simulink model "RejectDoublePress_Adhoc_Harness"  (R2019a)
settings: Solver=FixedStepDiscrete  StartTime=0.0  StopTime=Inf  FixedStep=0.1  RelTol=1e-3  EnableMultiTasking=on
settings Model: EnablePacing=on  Creator=colosky  LastModifiedBy=colosky
settings DataIOCC: LimitDataPoints=on  SaveFormat=Array  SaveOutput=off  SignalLogging=off  DSMLogging=off  SaveTime=off  ReturnWorkspaceOutputs=off
settings OptimizationCC: DefaultParameterBehavior=Inlined  InlineInvariantSignals=on  ExpressionDepthLimit=2147483647  InitFltsAndDblsToZero=on  NoFixptDivByZeroProtection=on  LifeSpan=inf
settings DebuggingCC: SignalInfNanChecking=warning  SaveWithParameterizedLinksMsg=none  UnderspecifiedInitializationDetection=Classic  MergeDetectMultiDrivingBlocksExec=none  SolverPrmCheckMsg=warning  FcnCallInpInsideContextMsg=warning  UniqueDataStoreMsg=warning  AllowSymbolicDim=off  StateNameClashWarn=warning  StrictBusMsg=ErrorOnBusTreatedAsVector  SFUnexpectedBacktrackingDiag=warning  SFNoUnconditionalDefaultTransitionDiag=warning  SFExecutionAtInitializationDiag=none  ArithmeticOperatorsInVariantConditions=warning
settings HardwareCC: ProdBitPerPointer=32  ProdBitPerSizeT=32  ProdBitPerPtrDiffT=32  ProdLargestAtomicFloat=None  ProdIntDivRoundTo=Undefined  ProdEndianess=Unspecified  ProdWordSize=32  ProdHWDeviceType=32-bit Generic
settings ModelReferenceCC: ModelReferenceNumInstancesAllowed=Single  PropagateSignalLabelsOutOfModel=off
settings SFSimCC: SimUseLocalCustomCode=off  SimParseCustomCode=off  MATLABDynamicMemAlloc=off
settings RTWCC: SystemTargetFile=ert.tlc  TemplateMakefile=ert_default_tmf  GenerateReport=on  RTWUseLocalCustomCode=off  IncludeHyperlinkInReport=on  LaunchReport=on  PortableWordSizes=on  GenerateTraceInfo=on  GenerateTraceReport=on  GenerateTraceReportSl=on  GenerateTraceReportSf=on  GenerateTraceReportEml=on
settings CodeAppCC: IgnoreCustomStorageClasses=off  CustomSymbolStrGlobalVar=$N$M  StateflowObjectComments=on
settings ERTTargetCC: MultiwordLength=2048  GenerateSampleERTMain=on  InlinedParameterPlacement=NonHierarchical  ERTCustomFileTemplate=example_file_process.tlc  ConvertIfToSwitch=off  SuppressUnreachableDefaultCases=off
settings ConfigComp: CovScope=ReferencedModels  CovMetricSettings=dcme  CovExternalEMLEnable=off  CovSFcnEnable=off  DVMode=DesignErrorDetection  DVMaxProcessTime=3000  DVDisplayUnsatisfiableObjectives=on  DVAutomaticStubbing=off  DVMakeOutputFilesUnique=off  DVParameters=on  DVParametersUseConfig=on  DVModelCoverageObjectives=MCDC  DVMaxTestCaseSteps=500  DVTestSuiteOptimization=CombinedObjectives  DVAssertions=EnableAll  DVProofAssumptions=EnableAll  DVIgnoreCovSatisfied=on  DVCoverageDataFile=CruiseControlCovManual.cvt  DVDetectDeadLogic=on  DVDetectActiveLogic=on  DVDetectIntegerOverflow=off  DVMaxViolationSteps=50  DVSaveDataFile=off  DVSaveHarnessModel=on  DVHarnessModelFileName=$ModelName$_harness_SLDV  DVReportIncludeGraphics=on  DVRebuildModelRepresentation=Always  PSAutoStubLUT=off

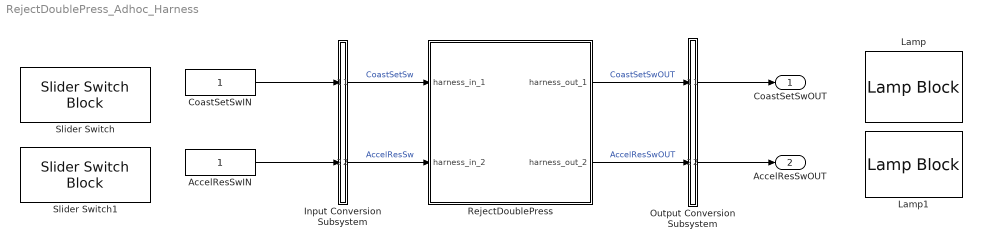
== system RejectDoublePress_Adhoc_Harness ==
  AccelResSwIN : Constant  OutDataTypeStr=boolean
  CoastSetSwIN : Constant  OutDataTypeStr=boolean
  Input Conversion Subsystem : Subsystem  Tag=__SLT_ICS__
  Lamp : LampBlock
  Lamp1 : LampBlock
  Output Conversion Subsystem : Subsystem  Tag=__SLT_OCS__
  RejectDoublePress : Subsystem  Tag=__SL_testing_harness_stub_
  Slider Switch : SliderSwitchBlock
      settings: Values={{'Off', 'On'}, [0 1]}
  Slider Switch1 : SliderSwitchBlock
      settings: Values={{'Off', 'On'}, [0 1]}
  CoastSetSwOUT : Outport  OutDataTypeStr=boolean  PortDimensions=[1]
  AccelResSwOUT : Outport  Port=2  OutDataTypeStr=boolean  PortDimensions=[1]
  wires:
  CoastSetSwIN/1 -> Input Conversion Subsystem/1(In_1)
  AccelResSwIN/1 -> Input Conversion Subsystem/2(In_2)
  Input Conversion Subsystem/1(Out_1) -> RejectDoublePress/1(harness_in_1)  "CoastSetSw"
  Input Conversion Subsystem/2(Out_2) -> RejectDoublePress/2(harness_in_2)  "AccelResSw"
  Output Conversion Subsystem/1(Out_1) -> CoastSetSwOUT/1
  Output Conversion Subsystem/2(Out_2) -> AccelResSwOUT/1
  RejectDoublePress/1(harness_out_1) -> Output Conversion Subsystem/1(In_1)  "CoastSetSwOUT"
  RejectDoublePress/2(harness_out_2) -> Output Conversion Subsystem/2(In_2)  "AccelResSwOUT"

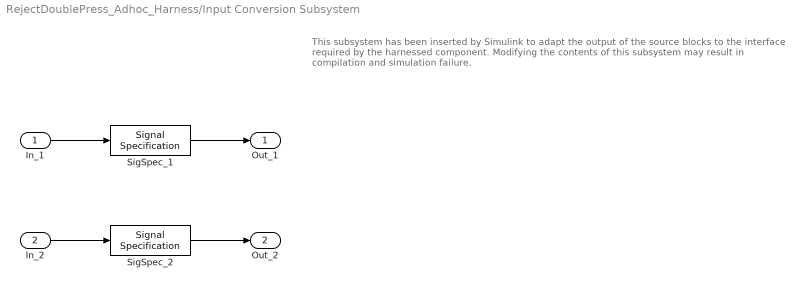
== system RejectDoublePress_Adhoc_Harness/Input Conversion Subsystem ==
  note: This subsystem has been inserted by Simulink to adapt the output of the source blocks to the interface required by the harnessed component.
      |  Modifying the contents of this subsystem may result in compilation and simulation failure.
  In_1 : Inport
  In_2 : Inport  Port=2
  SigSpec_1 : SignalSpecification  OutDataTypeStr=boolean  Dimensions=[1]  SampleTime=0.1
  SigSpec_2 : SignalSpecification  OutDataTypeStr=boolean  Dimensions=[1]  SampleTime=0.1
  Out_1 : Outport
  Out_2 : Outport  Port=2
  wires:
  In_1/1 -> SigSpec_1/1
  In_2/1 -> SigSpec_2/1
  SigSpec_1/1 -> Out_1/1
  SigSpec_2/1 -> Out_2/1

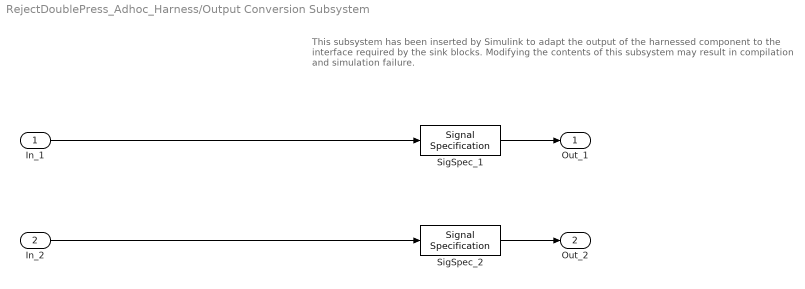
== system RejectDoublePress_Adhoc_Harness/Output Conversion Subsystem ==
  note: This subsystem has been inserted by Simulink to adapt the output of the harnessed component to the interface required by the sink blocks.
      |  Modifying the contents of this subsystem may result in compilation and simulation failure.
  In_1 : Inport
  In_2 : Inport  Port=2
  SigSpec_1 : SignalSpecification  OutDataTypeStr=boolean  Dimensions=[1]  SampleTime=0.1
  SigSpec_2 : SignalSpecification  OutDataTypeStr=boolean  Dimensions=[1]  SampleTime=0.1
  Out_1 : Outport
  Out_2 : Outport  Port=2
  wires:
  SigSpec_1/1 -> Out_1/1
  SigSpec_2/1 -> Out_2/1
  In_1/1 -> SigSpec_1/1
  In_2/1 -> SigSpec_2/1

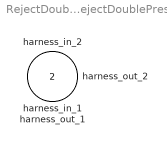
== system RejectDoublePress_Adhoc_Harness/RejectDoublePress ==
  harness_in_1 : Inport
  harness_in_2 : Inport  Port=2
  harness_out_1 : Outport
  harness_out_2 : Outport  Port=2
